simulink model "sampleModel1458"  (R2023a)
settings: Solver=VariableStepAuto  StartTime=0.0  StopTime=10.0  RelTol=1e-3
libraries: hdlsllib x5, simulink x3
settings Model: Creator=user1  LastModifiedBy=user1

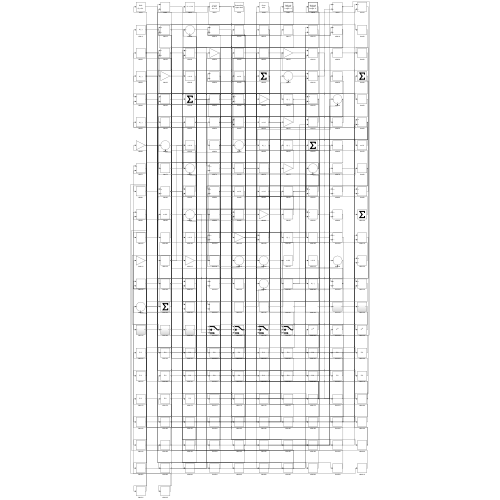
[thumbnail: Simulink's stored preview of the top-level diagram]
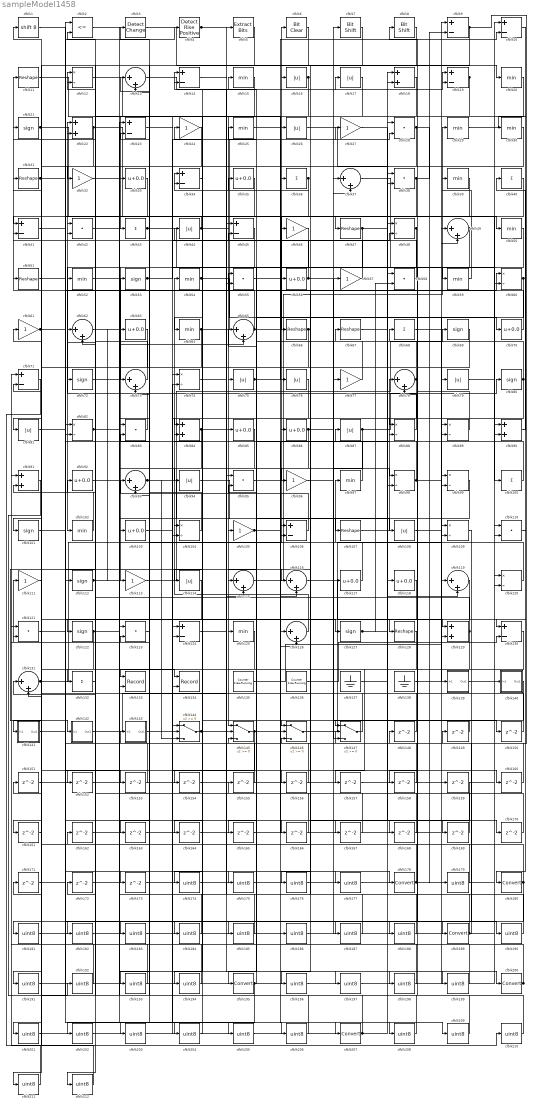
== system sampleModel1458 ==
  cfblk1 : ArithShift  BitShiftNumber=8
  cfblk{9..10,14,19,23,34,41,45,71,106,124,130} (12 alike) : Sum  Inputs=+-
  cfblk{36,40,43,68,100,132} (6 alike) : Sum  Inputs=+
  cfblk{21,53,69,72,80,101,112,122,127} (9 alike) : Signum
  cfblk{15,20,25,29..30,39,50,52,54,59,64,97,102,125} (14 alike) : MinMax
  cfblk{33,35,56,63,70,85..86,92,103,117..118} (11 alike) : Bias  Bias=0.0  SaturateOnIntegerOverflow=off
  cfblk{12,48,60,74,82,88..89,98..99,104,109,120} (12 alike) : Product  Inputs=*/  RndMeth=Zero  SaturateOnIntegerOverflow=on
  cfblk{24,27,32,46,57,61,77,96,105,111,113} (11 alike) : Gain
  cfblk{11,31,47,51,66..67,107,128} (8 alike) : Reshape
  cfblk{16..17,26,44,75..76,79,81,87,94,108,114} (12 alike) : Abs  SaturateOnIntegerOverflow=off
  cfblk{28,38,42,55,58,83,95,110,121,123} (10 alike) : DotProduct  OutDataTypeStr=Inherit: Inherit via internal rule
  cfblk{13,37,49,62,65,73,78,93,115..116,119,126,131} (13 alike) : Sum  Inputs=|++
  cfblk{18,22,84,90..91,129} (6 alike) : Sum
  cfblk133 : Record  FileSettingsInternal="{\"entries\":[{\"content\":{\"excelSettings\":{\"content\":{},\"type\":\"Streamout.ExcelSettings\"}},\"type\":\"Streamout.FileSettingStorage\",\"uuid\":\"\"}],\"packageUris\":[\"http:\\/\\/schema.mathworks.com\\/mf0\\/streamout_blocks\\/R2020a\"],\"version\":\"1.0\"}"  Layout=[1 1]  SignalsInternal="{\"entries\":[{\"content\":{\"signals\":[{\"content\":{\"blockPath\":[],\"dimensions\":[1],\"domain\":\"\",\"lineColor\":\"#a2142f\",\"plots\":[1],\"port\":1,\"signalID\":828,\"signalName\":\"XY Graph:1\"},\"type\":\"RecordBlkView.Signal\",\"uuid\":\"\"},{\"content\":{\"blockPath\":[],\"dimensions\":[1],\"domain\":\"\",\"lineColor\":\"#139fff\",\"plots\":[1],\"port\":2,\"signalID\":831,\"signalName\":\"XY Graph:2\"},\"type\":\"RecordBlkView.Signal\",\"uuid\":\"\"}]},\"type\":\"RecordBlkView.InputSignals\",\"uuid\":\"\"}],\"packageUris\":[\"http:\\/\\/schema.mathworks.com\\/mf0\\/streamout_blocks\\/R2020a\"],\"version\":\"1.0\"}"  VisualizationBindings="{\"xyplotplugin\":{\"info\":[{\"series\":[{\"bindingParametersList\":[{\"parameter\":\"X-Axis\",\"signalID\":828,\"signalName\":\"XY Graph:1\"},{\"parameter\":\"Y-Axis\",\"signalID\":831,\"signalName\":\"XY Graph:2\"}],\"seriesID\":39411}],\"subplotID\":1}]}}"  CompatibilityTag=XY  st=-1
  cfblk134 : Record  FileSettingsInternal="{\"entries\":[{\"content\":{\"excelSettings\":{\"content\":{},\"type\":\"Streamout.ExcelSettings\"}},\"type\":\"Streamout.FileSettingStorage\",\"uuid\":\"\"}],\"packageUris\":[\"http:\\/\\/schema.mathworks.com\\/mf0\\/streamout_blocks\\/R2020a\"],\"version\":\"1.0\"}"  Layout=[1 1]  SignalsInternal="{\"entries\":[{\"content\":{\"signals\":[{\"content\":{\"blockPath\":[],\"dimensions\":[1],\"domain\":\"\",\"lineColor\":\"#a2142f\",\"plots\":[1],\"port\":1,\"signalID\":836,\"signalName\":\"XY Graph:1\"},\"type\":\"RecordBlkView.Signal\",\"uuid\":\"\"},{\"content\":{\"blockPath\":[],\"dimensions\":[1],\"domain\":\"\",\"lineColor\":\"#139fff\",\"plots\":[1],\"port\":2,\"signalID\":839,\"signalName\":\"XY Graph:2\"},\"type\":\"RecordBlkView.Signal\",\"uuid\":\"\"}]},\"type\":\"RecordBlkView.InputSignals\",\"uuid\":\"\"}],\"packageUris\":[\"http:\\/\\/schema.mathworks.com\\/mf0\\/streamout_blocks\\/R2020a\"],\"version\":\"1.0\"}"  VisualizationBindings="{\"xyplotplugin\":{\"info\":[{\"series\":[{\"bindingParametersList\":[{\"parameter\":\"X-Axis\",\"signalID\":836,\"signalName\":\"XY Graph:1\"},{\"parameter\":\"Y-Axis\",\"signalID\":839,\"signalName\":\"XY Graph:2\"}],\"seriesID\":23982}],\"subplotID\":1}]}}"  CompatibilityTag=XY  st=-1
  cfblk135 : hdlsllib/Sources/Counter Free-Running  NumBits=16  tsamp=-1
  cfblk136 : hdlsllib/Sources/Counter Free-Running  NumBits=16  tsamp=-1
  cfblk137 : Ground
  cfblk138 : Ground
  cfblk139 : Subsystem
      settings: LibrarySourceBlock=|
      | hdlsllib/Ports &
      | Subsystems/Subsystem
  cfblk140 : Subsystem
      settings: LibrarySourceBlock=|
      | hdlsllib/Ports &
      | Subsystems/Subsystem
  cfblk141 : Subsystem
      settings: LibrarySourceBlock=|
      | hdlsllib/Ports &
      | Subsystems/Subsystem
  cfblk142 : Subsystem
      settings: LibrarySourceBlock=|
      | hdlsllib/Ports &
      | Subsystems/Subsystem
  cfblk143 : Subsystem
      settings: LibrarySourceBlock=|
      | hdlsllib/Ports &
      | Subsystems/Subsystem
  cfblk{144..147} (4 alike) : Switch  SaturateOnIntegerOverflow=off  InputSameDT=off
  cfblk{148..173} (26 alike) : Delay  SampleTime=1
  cfblk{174..177,179,181..188,190..194,196..199,201..206,208..212} (33 alike) : DataTypeConversion  OutDataTypeStr=uint8  SaturateOnIntegerOverflow=off  RndMeth=Floor
  cfblk{178,180,189,195,200,207} (6 alike) : DataTypeConversion  SaturateOnIntegerOverflow=off  RndMeth=Floor
  cfblk2 : RelationalOperator  Operator=<=  OutDataTypeStr=boolean  InputSameDT=off
  cfblk3 : simulink/Logic and Bit Operations/Detect Change  vinit=0  OutDataTypeStr=boolean
      settings: LibrarySourceBlock=|
      | hdlsllib/Logic and Bit
      | Operations/Detect
      | Change
  cfblk4 : hdlsllib/Logic and Bit Operations/Detect Rise Positive  vinit=0  OutDataTypeStr=boolean
  cfblk5 : simulink/Logic and Bit Operations/Extract Bits  bitsToExtract=Upper half  numBits=8  bitIdxRange=[0 7]  outScalingMode=Preserve fixed-point scaling
      settings: LibrarySourceBlock=|
      | hdlsllib/Logic and Bit
      | Operations/Extract Bits
  cfblk6 : simulink/Logic and Bit Operations/Bit Clear  iBit=0
      settings: LibrarySourceBlock=|
      | hdlsllib/Logic and Bit
      | Operations/Bit Clear
  cfblk7 : hdlsllib/Logic and Bit Operations/Bit Shift  mode=Shift Left Logical  N=0
  cfblk8 : hdlsllib/Logic and Bit Operations/Bit Shift  mode=Shift Left Logical  N=0
  wires:
  cfblk57/1 -> cfblk22/1
  cfblk110/1 -> cfblk180/1
  cfblk87/1 -> cfblk80/1, cfblk19/1, cfblk94/1
  cfblk15/1 -> cfblk43/1
  cfblk46/1 -> cfblk102/1
  cfblk115/1 -> cfblk29/1
  cfblk44/1 -> cfblk6/1, cfblk41/1
  cfblk66/1 -> cfblk111/1, cfblk131/2
  cfblk65/1 -> cfblk11/1, cfblk10/2
  cfblk63/1 -> cfblk142/1(In1)
  cfblk50/1 -> cfblk113/1
  cfblk83/1 -> cfblk42/1
  cfblk131/1 -> cfblk26/1, cfblk168/1
  cfblk5/1 -> cfblk52/1
  cfblk21/1 -> cfblk100/1, cfblk47/1
  cfblk22/1 -> cfblk66/1, cfblk32/1
  cfblk126/1 -> cfblk54/1
  cfblk16/1 -> cfblk145/1, cfblk114/1
  cfblk11/1 -> cfblk74/1
  cfblk129/1 -> cfblk131/1, cfblk62/2
  cfblk53/1 -> cfblk28/2, cfblk106/2
  cfblk132/1 -> cfblk92/1
  cfblk73/1 -> cfblk21/1
  cfblk7/1 -> cfblk46/1
  cfblk17/1 -> cfblk72/1
  cfblk58/1 -> cfblk12/1
  cfblk29/1 -> cfblk128/1
  cfblk23/1 -> cfblk207/1
  cfblk88/1 -> cfblk2/2
  cfblk78/1 -> cfblk75/1, cfblk116/1, cfblk34/1, cfblk73/1
  cfblk112/1 -> cfblk63/1, cfblk204/1
  cfblk60/1 -> cfblk185/1, cfblk188/1, cfblk196/1
  cfblk38/1 -> cfblk82/2, cfblk9/2
  cfblk68/1 -> cfblk139/1(In1)
  cfblk33/1 -> cfblk101/1
  cfblk56/1 -> cfblk3/1, cfblk98/1, cfblk98/2
  cfblk96/1 -> cfblk37/1
  cfblk12/1 -> cfblk126/1
  cfblk104/1 -> cfblk51/1
  cfblk117/1 -> cfblk97/1
  cfblk97/1 -> cfblk25/1
  cfblk72/1 -> cfblk53/1
  cfblk100/1 -> cfblk76/1
  cfblk86/1 -> cfblk133/2, cfblk150/1
  cfblk10/1 -> cfblk130/1
  cfblk116/1 -> cfblk129/1
  cfblk102/1 -> cfblk31/1
  cfblk47/1 -> cfblk170/1, cfblk212/1
  cfblk77/1 -> cfblk14/1
  cfblk122/1 -> cfblk62/1, cfblk161/1, cfblk177/1
  cfblk19/1 -> cfblk154/1, cfblk193/1
  cfblk34/1 -> cfblk64/1
  cfblk147/1 -> cfblk56/1
  cfblk20/1 -> cfblk96/1
  cfblk120/1 -> cfblk13/1
  cfblk93/1 -> cfblk107/1, cfblk144/3
  cfblk137/1 -> cfblk118/1
  cfblk64/1 -> cfblk18/1, cfblk132/1, cfblk127/1
  cfblk67/1 -> cfblk18/2
  cfblk35/1 -> cfblk133/1
  cfblk146/1 -> cfblk49/1
  cfblk6/1 -> cfblk81/1
  cfblk135/1 -> cfblk49/2
  cfblk76/1 -> cfblk105/1
  cfblk111/1 -> cfblk61/1
  cfblk109/1 -> cfblk189/1
  cfblk36/1 -> cfblk122/1, cfblk34/2
  cfblk121/1 -> cfblk125/1
  cfblk124/1 -> cfblk200/1
  cfblk127/1 -> cfblk58/1, cfblk58/2
  cfblk106/1 -> cfblk93/1
  cfblk37/1 -> cfblk90/2
  cfblk94/1 -> cfblk117/1
  cfblk74/1 -> cfblk60/1
  cfblk13/1 -> cfblk17/1
  cfblk48/1 -> cfblk41/2, cfblk165/1
  cfblk99/1 -> cfblk195/1
  cfblk101/1 -> cfblk87/1
  cfblk113/1 -> cfblk69/1
  cfblk40/1 -> cfblk83/1
  cfblk54/1 -> cfblk59/1, cfblk89/2, cfblk84/1
  cfblk18/1 -> cfblk146/1
  cfblk84/1 -> cfblk14/2, cfblk104/2, cfblk190/1
  cfblk26/1 -> cfblk48/1
  cfblk119/1 -> cfblk141/1(In1)
  cfblk3/1 -> cfblk20/1
  cfblk80/1 -> cfblk134/2, cfblk67/1, cfblk164/1
  cfblk49/1 -> cfblk115/1, cfblk158/1
  cfblk143/1(Out1) -> cfblk178/1
  cfblk4/1 -> cfblk5/1, cfblk50/1
  cfblk90/1 -> cfblk40/1
  cfblk79/1 -> cfblk10/1
  cfblk89/1 -> cfblk8/1
  cfblk61/1 -> cfblk116/2, cfblk206/1
  cfblk25/1 -> cfblk70/1
  cfblk31/1 -> cfblk173/1, cfblk187/1
  cfblk107/1 -> cfblk78/1
  cfblk55/1 -> cfblk27/1
  cfblk82/1 -> cfblk134/1, cfblk108/1
  cfblk125/1 -> cfblk144/2
  cfblk70/1 -> cfblk15/1
  cfblk105/1 -> cfblk126/2, cfblk169/1
  cfblk62/1 -> cfblk103/1
  cfblk136/1 -> cfblk130/2
  cfblk145/1 -> cfblk88/2, cfblk181/1
  cfblk141/1(Out1) -> cfblk4/1
  cfblk81/1 -> cfblk55/1
  cfblk9/1 -> cfblk147/2, cfblk201/1
  cfblk142/1(Out1) -> cfblk85/1
  cfblk42/1 -> cfblk65/2
  cfblk59/1 -> cfblk39/1
  cfblk43/1 -> cfblk115/2, cfblk48/2, cfblk55/2
  cfblk118/1 -> cfblk147/3
  cfblk69/1 -> cfblk88/1
  cfblk98/1 -> cfblk119/1, cfblk35/1
  cfblk138/1 -> cfblk129/2
  cfblk1/1 -> cfblk112/1
  cfblk8/1 -> cfblk33/1
  cfblk28/1 -> cfblk146/2, cfblk179/1
  cfblk75/1 -> cfblk36/1, cfblk209/1
  cfblk27/1 -> cfblk119/2
  cfblk108/1 -> cfblk9/1
  cfblk144/1 -> cfblk16/1, cfblk104/1, cfblk19/2
  cfblk139/1(Out1) -> cfblk30/1
  cfblk148/1 -> cfblk28/1
  cfblk149/1 -> cfblk147/1
  cfblk150/1 -> cfblk121/1
  cfblk151/1 -> cfblk145/2
  cfblk130/1 -> cfblk152/1
  cfblk152/1 -> cfblk144/1
  cfblk51/1 -> cfblk153/1
  cfblk153/1 -> cfblk82/1
  cfblk154/1 -> cfblk60/2
  cfblk155/1 -> cfblk13/2
  cfblk14/1 -> cfblk156/1
  cfblk156/1 -> cfblk65/1
  cfblk128/1 -> cfblk157/1
  cfblk157/1 -> cfblk90/1
  cfblk158/1 -> cfblk146/3
  cfblk103/1 -> cfblk160/1
  cfblk160/1 -> cfblk83/2
  cfblk161/1 -> cfblk1/1
  cfblk162/1 -> cfblk74/2
  cfblk39/1 -> cfblk163/1
  cfblk163/1 -> cfblk106/1
  cfblk165/1 -> cfblk89/1
  cfblk41/1 -> cfblk166/1
  cfblk166/1 -> cfblk12/2
  cfblk52/1 -> cfblk167/1
  cfblk167/1 -> cfblk93/2
  cfblk168/1 -> cfblk42/2
  cfblk169/1 -> cfblk73/2
  cfblk170/1 -> cfblk78/2
  cfblk173/1 -> cfblk7/1
  cfblk140/1(Out1) -> cfblk174/1
  cfblk174/1 -> cfblk79/1
  cfblk2/1 -> cfblk175/1
  cfblk175/1 -> cfblk140/1(In1)
  cfblk159/1 -> cfblk176/1
  cfblk176/1 -> cfblk37/2
  cfblk177/1 -> cfblk159/1
  cfblk178/1 -> cfblk155/1, cfblk84/2, cfblk45/2, cfblk121/2
  cfblk179/1 -> cfblk143/1(In1)
  cfblk180/1 -> cfblk45/1, cfblk68/1, cfblk191/1
  cfblk181/1 -> cfblk110/1
  cfblk114/1 -> cfblk182/1
  cfblk182/1 -> cfblk110/2
  cfblk123/1 -> cfblk183/1
  cfblk183/1 -> cfblk57/1
  cfblk85/1 -> cfblk184/1
  cfblk184/1 -> cfblk123/1
  cfblk185/1 -> cfblk123/2
  cfblk95/1 -> cfblk186/1
  cfblk186/1 -> cfblk77/1
  cfblk187/1 -> cfblk95/1
  cfblk188/1 -> cfblk95/2
  cfblk189/1 -> cfblk149/1, cfblk86/1
  cfblk190/1 -> cfblk109/1
  cfblk191/1 -> cfblk109/2
  cfblk91/1 -> cfblk192/1
  cfblk192/1 -> cfblk151/1
  cfblk193/1 -> cfblk91/1
  cfblk45/1 -> cfblk194/1
  cfblk194/1 -> cfblk91/2
  cfblk195/1 -> cfblk145/3, cfblk120/2, cfblk202/1
  cfblk196/1 -> cfblk99/1
  cfblk164/1 -> cfblk197/1
  cfblk197/1 -> cfblk99/2
  cfblk172/1 -> cfblk198/1
  cfblk198/1 -> cfblk22/2
  cfblk32/1 -> cfblk199/1
  cfblk199/1 -> cfblk172/1
  cfblk200/1 -> cfblk44/1, cfblk120/1
  cfblk201/1 -> cfblk124/1
  cfblk202/1 -> cfblk124/2
  cfblk24/1 -> cfblk203/1
  cfblk203/1 -> cfblk38/1
  cfblk204/1 -> cfblk24/1
  cfblk171/1 -> cfblk205/1
  cfblk205/1 -> cfblk38/2
  cfblk206/1 -> cfblk171/1
  cfblk207/1 -> cfblk162/1, cfblk2/1
  cfblk92/1 -> cfblk208/1
  cfblk208/1 -> cfblk23/1
  cfblk209/1 -> cfblk23/2
  cfblk71/1 -> cfblk210/1
  cfblk210/1 -> cfblk148/1
  cfblk30/1 -> cfblk211/1
  cfblk211/1 -> cfblk71/1
  cfblk212/1 -> cfblk71/2

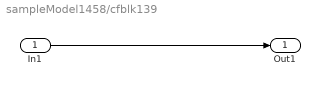
== system sampleModel1458/cfblk139 ==
  In1 : Inport
  Out1 : Outport
  wires:
  In1/1 -> Out1/1

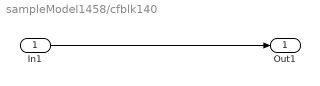
== system sampleModel1458/cfblk140 ==
  In1 : Inport
  Out1 : Outport
  wires:
  In1/1 -> Out1/1

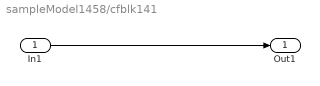
== system sampleModel1458/cfblk141 ==
  In1 : Inport
  Out1 : Outport
  wires:
  In1/1 -> Out1/1

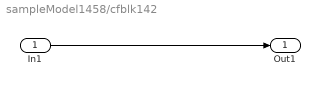
== system sampleModel1458/cfblk142 ==
  In1 : Inport
  Out1 : Outport
  wires:
  In1/1 -> Out1/1

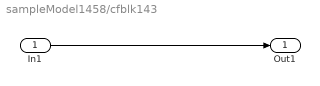
== system sampleModel1458/cfblk143 ==
  In1 : Inport
  Out1 : Outport
  wires:
  In1/1 -> Out1/1
